simulink model "verify_Simple_House_mdl"  (R2016b)
settings: Solver=ode45  StartTime=0  StopTime=365*24*3600  RelTol=1e-3  EnableMultiTasking=on
InitFcn:
  | load('DE_TRY2010_04_averageYear')
libraries: carnot x3
settings Model: Creator=drhf  LastModifiedBy=drhf
settings DataIOCC: SaveFormat=Array  SignalLoggingSaveFormat=ModelDataLogs
settings OptimizationCC: ExpressionDepthLimit=2147483647  LifeSpan=inf
settings DebuggingCC: UnderspecifiedInitializationDetection=Classic  MergeDetectMultiDrivingBlocksExec=none  SolverPrmCheckMsg=warning  FcnCallInpInsideContextMsg=warning  StateNameClashWarn=warning  SFUnexpectedBacktrackingDiag=warning  SFNoUnconditionalDefaultTransitionDiag=warning  SFExecutionAtInitializationDiag=none
settings HardwareCC: ProdBitPerPointer=32  ProdBitPerSizeT=32  ProdBitPerPtrDiffT=32  ProdLargestAtomicFloat=None  ProdIntDivRoundTo=Undefined  ProdEndianess=Unspecified  ProdWordSize=32  ProdHWDeviceType=32-bit Generic
settings ModelReferenceCC: PropagateSignalLabelsOutOfModel=off
settings GRTTargetCC: TargetLangStandard=C89/C90 (ANSI)  GeneratePreprocessorConditionals=Disable all  CombineOutputUpdateFcns=off  GRTInterface=on
settings ConfigComp: CovMetricSettings=dw  CovHtmlReporting=on  CovSaveCumulativeToWorkspaceVar=on  CovSaveSingleToWorkspaceVar=on  CovExternalEMLEnable=off

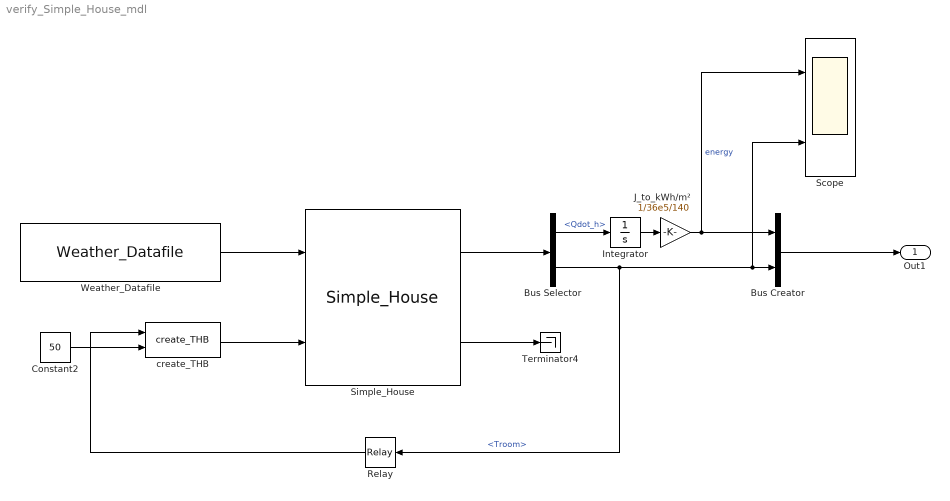
== system verify_Simple_House_mdl ==
  Bus Creator : BusCreator  Inputs=2
  Bus Selector : BusSelector  OutputSignals=Qdot.Qdot_h,Troom
  Constant2 : Constant  Value=50
  Integrator : Integrator
  J_to_kWh/m² : Gain  Gain=1/36e5/140
  Relay : Relay  OnSwitchValue=20.1  OffSwitchValue=19.9  OnOutputValue=0  OffOutputValue=800/3600
  Scope : Scope  NumInputPorts=2
  Simple_House : carnot/Load/Houses/Simple_House  Ahabit=140  Hroom=2.6  Floorsize=[7 10]  UAwall=0.162*(54.6+26.4)+0.182*((45.7+56.0)*2 -(12+4+3+4))  UAneighbour=0  Uground=0.18  mc=0.5e6*140 % 0.5 MJ/m2/K  shade=0.75  tini=20  Awin=[12 4 3 4]  AziWin=[0 90 -180 -90]  Uwin="[1    1   1    1]*1.0"  Gwin="[1    1   1    1]*0.585*(1-0.15)"  vent=0.4  rec=0.6  heatload=1792  dpcoeff=[10 100]  delta_t_nom=15  n_rad=1.1  mass_times_cap=40e6
  Terminator4 : Terminator
  Weather_Datafile : carnot/Weather/Weather_Datafile  PathName='C:\repos\carnot_svn\trunk\public\data\'  FileName='DE_TRY2010_04_averageYear.mat'  UserParam=off  VariableName=DE_TRY2010_04_averageYear  SampleTime=3600
  create_THB : carnot/Source/Simple/create_THB  p=1e5  fluid=Water  mix=0  mix2=0  mix3=0  dia=0.02  hgt=0  mID=No Pressure Drop
  Out1 : Outport
  wires:
  Weather_Datafile/1 -> Simple_House/1
  Bus Creator/1 -> Out1/1
  Simple_House/2 -> Terminator4/1
  Simple_House/1 -> Bus Selector/1
  Bus Selector/2 -> Relay/1, Bus Creator/2, Scope/2  "<Troom>"
  Constant2/1 -> create_THB/2
  Relay/1 -> create_THB/1
  create_THB/1 -> Simple_House/2
  Bus Selector/1 -> Integrator/1  "<Qdot_h>"
  Integrator/1 -> J_to_kWh/m²/1
  J_to_kWh/m²/1 -> Scope/1, Bus Creator/1  "energy"
